simulink model "SpeedgoatCANOpen2Buses1ms"  (R2018b)
settings: Solver=ode8  StartTime=0.0  StopTime=inf  FixedStep=0.001  RelTol=1e-3  EnableMultiTasking=on
undefined symbols (not defined in the file or in its folder): DiscIntNeverNeededParam
libraries: slrtlib x6, speedgoatlib_IO691 x5, dspstat3 x5, simulink x5
(part 2 of 3)

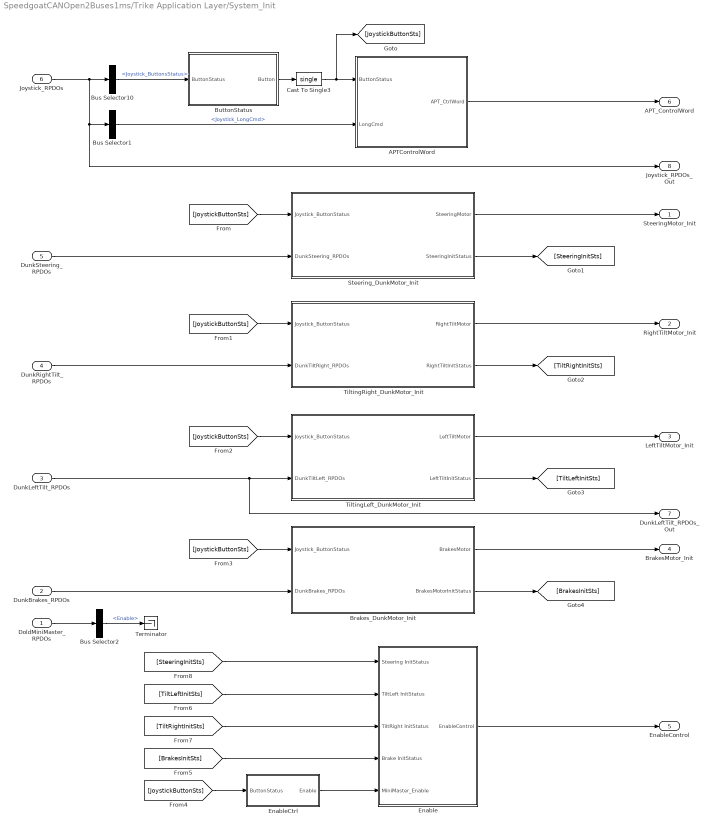
== system SpeedgoatCANOpen2Buses1ms/Trike Application Layer/System_Init ==
  DoldMiniMaster_RPDOs : Inport  OutDataTypeStr=Bus: Dold_RPDOs
  DunkBrakes_RPDOs : Inport  Port=2  OutDataTypeStr=Bus: Dunk_RPDOs
  DunkLeftTilt_RPDOs : Inport  Port=3  OutDataTypeStr=Bus: Dunk_RPDOs
  DunkRightTilt_RPDOs : Inport  Port=4  OutDataTypeStr=Bus: Dunk_RPDOs
  DunkSteering_RPDOs : Inport  Port=5  OutDataTypeStr=Bus: Dunk_RPDOs
  Joystick_RPDOs : Inport  Port=6  OutDataTypeStr=Bus: Joystick_RPDOs
  APTControlWord : MATLAB Function  TreatAsAtomicUnit=on
  Brakes_DunkMotor_Init : Subsystem
  Bus Selector1 : BusSelector  OutputSignals=Joystick_LongCmd
  Bus Selector10 : BusSelector  OutputSignals=Joystick_ButtonsStatus
  Bus Selector2 : BusSelector  OutputSignals=Enable
  ButtonStatus : MATLAB Function  TreatAsAtomicUnit=on
  Cast To Single3 : DataTypeConversion  OutDataTypeStr=single
  Enable : Subsystem
  EnableCtrl : Stateflow chart  TreatAsAtomicUnit=on
  Steering_DunkMotor_Init : Subsystem
  Terminator : Terminator
  TiltingLeft_DunkMotor_Init : Subsystem
  TiltingRight_DunkMotor_Init : Subsystem
  SteeringMotor_Init : Outport  OutDataTypeStr=Bus: Dunk_Init_TPDOs
  RightTiltMotor_Init : Outport  Port=2  OutDataTypeStr=Bus: Dunk_Init_TPDOs
  LeftTiltMotor_Init : Outport  Port=3  OutDataTypeStr=Bus: Dunk_Init_TPDOs
  BrakesMotor_Init : Outport  Port=4  OutDataTypeStr=Bus: DunkBrakes_Init_TPDOs
  EnableControl : Outport  Port=5
  APT_ControlWord : Outport  Port=6
  DunkLeftTilt_RPDOs_Out : Outport  Port=7  OutDataTypeStr=Bus: Dunk_RPDOs
  Joystick_RPDOs_Out : Outport  Port=8  OutDataTypeStr=Bus: Joystick_RPDOs
  wires:
  Bus Selector10/1 -> ButtonStatus/1(ButtonStatus)  "<Joystick_ButtonsStatus>"
  Joystick_RPDOs/1 -> Bus Selector10/1, Joystick_RPDOs_Out/1, Bus Selector1/1
  DunkBrakes_RPDOs/1 -> Brakes_DunkMotor_Init/2(DunkBrakes_RPDOs)
  DunkLeftTilt_RPDOs/1 -> TiltingLeft_DunkMotor_Init/2(DunkTiltLeft_RPDOs), DunkLeftTilt_RPDOs_Out/1
  DunkRightTilt_RPDOs/1 -> TiltingRight_DunkMotor_Init/2(DunkTiltRight_RPDOs)
  DunkSteering_RPDOs/1 -> Steering_DunkMotor_Init/2(DunkSteering_RPDOs)
  Steering_DunkMotor_Init/1(SteeringMotor) -> SteeringMotor_Init/1
  TiltingRight_DunkMotor_Init/1(RightTiltMotor) -> RightTiltMotor_Init/1
  TiltingLeft_DunkMotor_Init/1(LeftTiltMotor) -> LeftTiltMotor_Init/1
  Brakes_DunkMotor_Init/1(BrakesMotor) -> BrakesMotor_Init/1
  APTControlWord/1(APT_CtrlWord) -> APT_ControlWord/1
  Bus Selector1/1 -> APTControlWord/2(LongCmd)  "<Joystick_LongCmd>"
  ButtonStatus/1(Button) -> Cast To Single3/1
  Enable/1(EnableControl) -> EnableControl/1
  DoldMiniMaster_RPDOs/1 -> Bus Selector2/1
  EnableCtrl/1(Enable) -> Enable/5(MiniMaster_Enable)
  Bus Selector2/1 -> Terminator/1  "<Enable>"
  Cast To Single3/1 -> APTControlWord/1(ButtonStatus), [JoystickButtonSts]
  [JoystickButtonSts] -> Steering_DunkMotor_Init/1(Joystick_ButtonStatus)
  [JoystickButtonSts] -> TiltingRight_DunkMotor_Init/1(Joystick_ButtonStatus)
  [JoystickButtonSts] -> Brakes_DunkMotor_Init/1(Joystick_ButtonStatus)
  [JoystickButtonSts] -> TiltingLeft_DunkMotor_Init/1(Joystick_ButtonStatus)
  [JoystickButtonSts] -> EnableCtrl/1(ButtonStatus)
  [BrakesInitSts] -> Enable/4(Brake InitStatus)
  Brakes_DunkMotor_Init/2(BrakesMotorInitStatus) -> [BrakesInitSts]
  TiltingLeft_DunkMotor_Init/2(LeftTiltInitStatus) -> [TiltLeftInitSts]
  TiltingRight_DunkMotor_Init/2(RightTiltInitStatus) -> [TiltRightInitSts]
  Steering_DunkMotor_Init/2(SteeringInitStatus) -> [SteeringInitSts]
  [SteeringInitSts] -> Enable/1(Steering InitStatus)
  [TiltLeftInitSts] -> Enable/2(TiltLeft InitStatus)
  [TiltRightInitSts] -> Enable/3(TiltRight InitStatus)

== system SpeedgoatCANOpen2Buses1ms/Speedgoat_TPDOs/CAN Bus Communication/CANOpen Slave Protocol Stack - CAN Bus #1 (A) ==
  C Caller : CCaller  FunctionName=CANOpenSlave_ProcessStack  PortSpecificationStruct="%)30     .    ( D   8    (     @         %    \"     8    !     0         %  0 \"0    $    V    07)G3F%M90  4&]R=$YA;64 4V-O<&4     26YD97@     5'EP90      4VEZ90         .    ,     8    (    !          %    \"     $    $     0         0  0 <GA)1 X    P    !@    @    $          4    (     0    0    !         !  ! !R>$E$#@   #@    &    \"     0         !0    @    !    !0    $         $     4   !);G ...(+2763 chars)"
  CAN RX Wrapper : Subsystem
  CAN TX Wrapper : Subsystem
  wires:
  C Caller/2 -> CAN TX Wrapper/Enable, CAN TX Wrapper/2(DLC)
  CAN RX Wrapper/1(ID) -> C Caller/1
  C Caller/1 -> CAN TX Wrapper/1(ID)
  CAN RX Wrapper/2(DLC) -> C Caller/2
  C Caller/3 -> CAN TX Wrapper/3(DATA)
  CAN RX Wrapper/3(DATA) -> C Caller/3

== system SpeedgoatCANOpen2Buses1ms/Speedgoat_TPDOs/CAN Bus Communication/CANOpen Slave Protocol Stack - CAN Bus #2 (B) ==
  C Caller : CCaller  FunctionName=CANOpenSlave_ProcessStack_APT  PortSpecificationStruct="%)30     .    ( D   8    (     @         %    \"     8    !     0         %  0 \"0    $    V    07)G3F%M90  4&]R=$YA;64 4V-O<&4     26YD97@     5'EP90      4VEZ90         .    ,     8    (    !          %    \"     $    $     0         0  0 <GA)1 X    P    !@    @    $          4    (     0    0    !         !  ! !R>$E$#@   #@    &    \"     0         !0    @    !    !0    $         $     4   !);G ...(+2763 chars)"
  CAN RX Wrapper : Subsystem
  CAN TX Wrapper : Subsystem
  wires:
  CAN RX Wrapper/3(DATA) -> C Caller/3
  C Caller/3 -> CAN TX Wrapper/3(DATA)
  CAN RX Wrapper/2(DLC) -> C Caller/2
  C Caller/1 -> CAN TX Wrapper/1(ID)
  CAN RX Wrapper/1(ID) -> C Caller/1
  C Caller/2 -> CAN TX Wrapper/2(DLC), CAN TX Wrapper/Enable

== system SpeedgoatCANOpen2Buses1ms/Trike Application Layer/System_Control/BrakeControl ==
  VehSpeed_SI [m/s] : Inport
  DriverBrakingRequest : Inport  Port=2
  Joystick_LongCmd : Inport  Port=3
  Joystick_ButtonStatus : Inport  Port=4
  BrakesMotor_CurrentInit : Inport  Port=5
  BrakeCtrlIn : Inport  Port=6
  Cast To Single3 : DataTypeConversion  Commented=on  OutDataTypeStr=single
  DecisionBrakeCtrl : Stateflow chart  TreatAsAtomicUnit=on
  Gain4 : Gain  Commented=on  Gain=0.001
  Gain5 : Gain  Gain=-1
  MATLAB Function : MATLAB Function  Commented=on  TreatAsAtomicUnit=on
  Subsystem : Subsystem
  Sum4 : Sum  Inputs=|++
  BrakesMotor_CurrentReq [mA] : Outport
  BrakesMotor_BrakeCtrl : Outport  Port=2
  wires:
  Joystick_LongCmd/1 -> DecisionBrakeCtrl/5(JsLongCmd)
  MATLAB Function/1(button) -> Cast To Single3/1
  Joystick_ButtonStatus/1 -> DecisionBrakeCtrl/4(JsButton)
  Cast To Single3/1 -> Gain4/1
  BrakesMotor_CurrentInit/1 -> Gain5/1
  Gain5/1 -> Sum4/1  "BrakesMotor_CurrentInit [mA]"
  Sum4/1 -> BrakesMotor_CurrentReq [mA]/1
  BrakeCtrlIn/1 -> DecisionBrakeCtrl/3(BrakeCtrlIn)
  DecisionBrakeCtrl/2(BrakeCtrl) -> BrakesMotor_BrakeCtrl/1
  DriverBrakingRequest/1 -> Subsystem/1(BrakingRequest)  "BrakingRequest [LSB]"
  Subsystem/1(BrakesMotor_CurrentReq) -> DecisionBrakeCtrl/1(BrakesMotor_CurrentReqIn)
  VehSpeed_SI [m/s]/1 -> DecisionBrakeCtrl/2(VehSpeed)
  DecisionBrakeCtrl/1(BrakesMotor_CurrentReq) -> Sum4/2  "Retract_current"

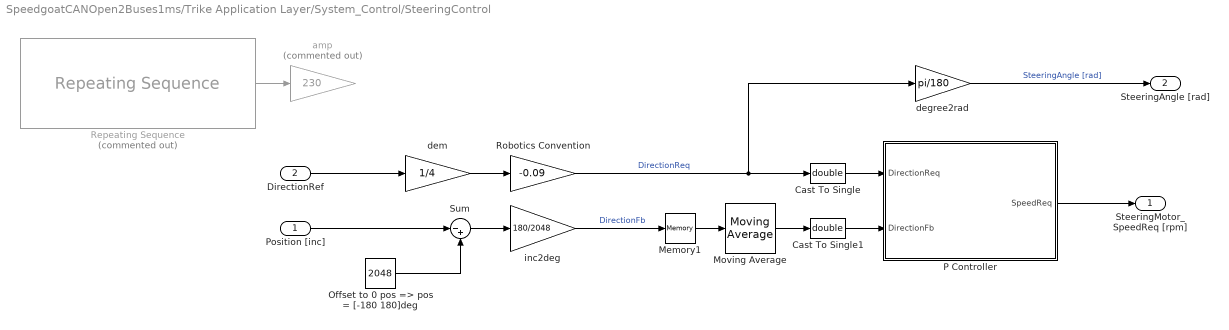
== system SpeedgoatCANOpen2Buses1ms/Trike Application Layer/System_Control/SteeringControl ==
  Position [inc] : Inport
  DirectionRef : Inport  Port=2
  Cast To Single : DataTypeConversion  OutDataTypeStr=double
  Cast To Single1 : DataTypeConversion  OutDataTypeStr=double
  Memory1 : Memory  InheritSampleTime=on
  Moving Average : dspstat3/Moving Average  Method=Sliding window  ForgettingFactorPort=off  SpecifyWindowLength=on  WindowLength=1  ForgettingFactor=0.9  SimulateUsing=Code generation
  Offset to 0 pos => pos = [-180 180]deg : Constant  Value=2048
  P Controller : MATLAB Function  TreatAsAtomicUnit=on  SystemSampleTime=5e-3
  Repeating Sequence : simulink/Sources/Repeating Sequence  Commented=on  rep_seq_t=[0 3 3.01 6 6.01 9 9.01 12]*5  rep_seq_y=[1 1 0 0 -1 -1 0 0]
  Robotics Convention : Gain  Gain=-0.09
  Sum : Sum  Inputs=|-+
  amp : Gain  Commented=on  Gain=230
  degree2rad : Gain  Gain=pi/180
  dem : Gain  Gain=1/4
  inc2deg : Gain  Gain=180/2048
  SteeringMotor_SpeedReq [rpm] : Outport
  SteeringAngle [rad] : Outport  Port=2
  wires:
  Memory1/1 -> Moving Average/1
  degree2rad/1 -> SteeringAngle [rad]/1  "SteeringAngle [rad]"
  inc2deg/1 -> Memory1/1  "DirectionFb"
  DirectionRef/1 -> dem/1
  P Controller/1(SpeedReq) -> SteeringMotor_SpeedReq [rpm]/1
  Robotics Convention/1 -> Cast To Single/1, degree2rad/1  "DirectionReq"
  Cast To Single/1 -> P Controller/1(DirectionReq)
  Cast To Single1/1 -> P Controller/2(DirectionFb)
  Position [inc]/1 -> Sum/1
  Sum/1 -> inc2deg/1
  Offset to 0 pos => pos = [-180 180]deg/1 -> Sum/2
  Moving Average/1 -> Cast To Single1/1
  Repeating Sequence/1 -> amp/1
  dem/1 -> Robotics Convention/1

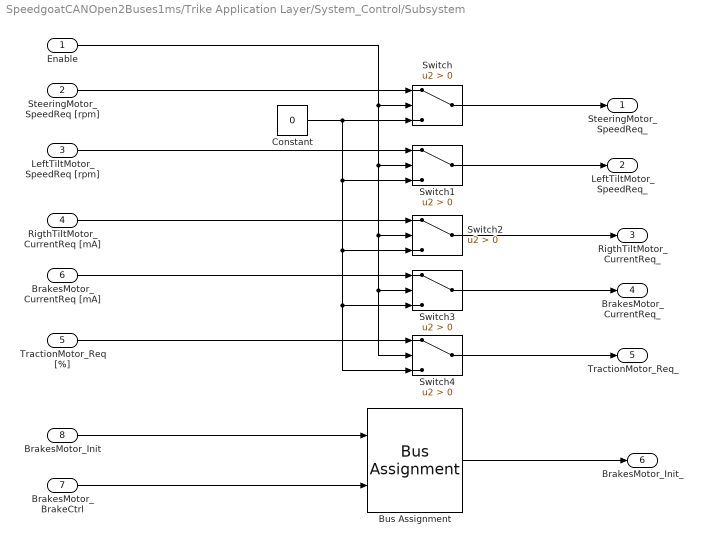
== system SpeedgoatCANOpen2Buses1ms/Trike Application Layer/System_Control/Subsystem ==
  Enable : Inport
  SteeringMotor_SpeedReq [rpm] : Inport  Port=2
  LeftTiltMotor_SpeedReq [rpm] : Inport  Port=3
  RigthTiltMotor_CurrentReq [mA] : Inport  Port=4
  TractionMotor_Req [%] : Inport  Port=5
  BrakesMotor_CurrentReq [mA] : Inport  Port=6
  BrakesMotor_BrakeCtrl : Inport  Port=7
  BrakesMotor_Init : Inport  Port=8  OutDataTypeStr=Bus: DunkBrakes_Init_TPDOs
  Bus Assignment : BusAssignment  AssignedSignals=BrakeCtrl
  Constant : Constant  Value=0
  Switch{,1..4} (5 alike) : Switch  Criteria=u2 > Threshold
  SteeringMotor_SpeedReq_ : Outport
  LeftTiltMotor_SpeedReq_ : Outport  Port=2
  RigthTiltMotor_CurrentReq_ : Outport  Port=3
  BrakesMotor_CurrentReq_ : Outport  Port=4
  TractionMotor_Req_ : Outport  Port=5
  BrakesMotor_Init_ : Outport  Port=6  OutDataTypeStr=Bus: DunkBrakes_Init_TPDOs
  wires:
  TractionMotor_Req [%]/1 -> Switch4/1
  Switch1/1 -> LeftTiltMotor_SpeedReq_/1
  Switch2/1 -> RigthTiltMotor_CurrentReq_/1
  Enable/1 -> Switch1/2, Switch2/2, Switch3/2, Switch4/2, Switch/2
  SteeringMotor_SpeedReq [rpm]/1 -> Switch/1
  LeftTiltMotor_SpeedReq [rpm]/1 -> Switch1/1
  Constant/1 -> Switch3/3, Switch4/3, Switch2/3, Switch1/3, Switch/3
  Switch/1 -> SteeringMotor_SpeedReq_/1
  BrakesMotor_CurrentReq [mA]/1 -> Switch3/1
  Switch3/1 -> BrakesMotor_CurrentReq_/1
  Switch4/1 -> TractionMotor_Req_/1
  RigthTiltMotor_CurrentReq [mA]/1 -> Switch2/1
  Bus Assignment/1 -> BrakesMotor_Init_/1
  BrakesMotor_Init/1 -> Bus Assignment/1
  BrakesMotor_BrakeCtrl/1 -> Bus Assignment/2

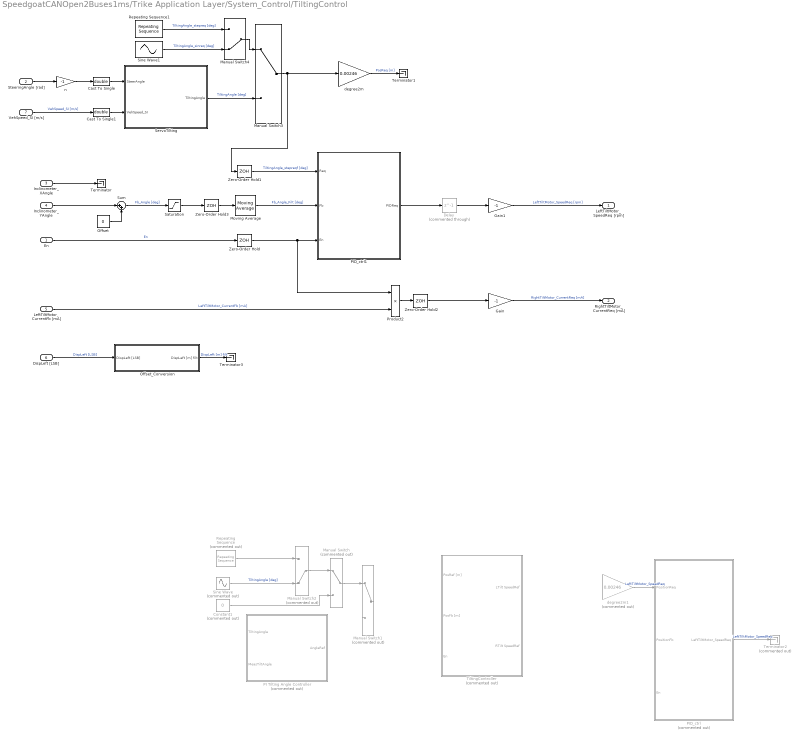
== system SpeedgoatCANOpen2Buses1ms/Trike Application Layer/System_Control/TiltingControl ==
  En : Inport
  SteeringAngle [rad] : Inport  Port=2
  Inclinometer_XAngle : Inport  Port=3
  Inclinometer_YAngle : Inport  Port=4
  LeftTiltMotor_CurrentFb [mA] : Inport  Port=5
  DispLeft [LSB] : Inport  Port=6
  VehSpeed_SI [m/s] : Inport  Port=7
  Cast To Single : DataTypeConversion  OutDataTypeStr=double
  Cast To Single1 : DataTypeConversion  OutDataTypeStr=double
  Constant1 : Constant  Commented=on  Value=0
  Delay : Delay  Commented=through  DelayLength=1  SampleTime=0.005
  Gain : Gain  Gain=-1
  Gain1 : Gain  Gain=-1
  Manual Switch : ManualSwitch  Commented=on
  Manual Switch1 : ManualSwitch  Commented=on
  Manual Switch2 : ManualSwitch  Commented=on  CurrentSetting=0
  Manual Switch3 : ManualSwitch
  Manual Switch4 : ManualSwitch  CurrentSetting=0
  Moving Average : dspstat3/Moving Average  Method=Sliding window  ForgettingFactorPort=off  SpecifyWindowLength=on  WindowLength=10  ForgettingFactor=0.9  SimulateUsing=Code generation
  Offset : Constant  Value=0
  Offset_Conversion : Subsystem
  PI Tilting Angle Controller : Subsystem  Commented=on  TreatAsAtomicUnit=on  SystemSampleTime=10e-3
  PID_ctrl : Subsystem  Commented=on  mask{Kp=80000, Ki=200, Kd=0, Ts=0.005, N=1, FF_En=0, Req_lim=2000}
      mask prompts: N "FilterOrder"; FF_En "FeedForward En"; Req_lim "Req_sat"
  PID_ctrl1 : Subsystem  mask{Kp=90, Ki=0, Kd=2, Ts=0.015, N=4, FF_En=0, Req_lim=1000}
      mask prompts: N "FilterOrder"; FF_En "FeedForward En"; Req_lim "Req_sat"
  Product2 : Product
  Repeating Sequence : simulink/Sources/Repeating Sequence  Commented=on  rep_seq_t=[0 3 3.01 6 6.01 9 9.01 12]*5  rep_seq_y=[ 0 0 1 1 0 0 1 1]*3
  Repeating Sequence1 : simulink/Sources/Repeating Sequence  rep_seq_t=[0 3 3.001 6 6.001 9 9.001 12] * 4 + 50  rep_seq_y=[ 0 0 1 1 0 0 -1 -1]*2
  Saturation : Saturate  UpperLimit=30  LowerLimit=-30
  ServoTilting : MATLAB Function  TreatAsAtomicUnit=on
      settings: MinAlgLoopOccurrences=on
  Sine Wave : Sin  Commented=on  Amplitude=2  Frequency=0.5  SampleTime=0
  Sine Wave1 : Sin  Amplitude=2  Frequency=0.5  SampleTime=0
  Sum : Sum  Inputs=|++
  Terminator : Terminator
  Terminator1 : Terminator
  Terminator2 : Terminator  Commented=on
  Terminator3 : Terminator
  TiltingController : Subsystem  Commented=on  VariantControlMode=Label  Variant=on  VariantControl=Variant1  LabelModeActiveChoice=V1  PropagateVariantConditions=on
  Zero-Order Hold{,1..3} (4 alike) : ZeroOrderHold  SampleTime=0.005
  degree2m : Gain  Gain=0.00246
  degree2m1 : Gain  Commented=on  Gain=0.00246
  n : Gain  Gain=-1
  LeftTiltMotor_SpeedReq [rpm] : Outport
  RightTiltMotor_CurrentReq [mA] : Outport  Port=2
  wires:
  SteeringAngle [rad]/1 -> n/1
  Cast To Single/1 -> ServoTilting/1(SteerAngle)
  Cast To Single1/1 -> ServoTilting/2(VehSpeed_SI)
  VehSpeed_SI [m/s]/1 -> Cast To Single1/1  "VehSpeed_SI [m/s]"
  Constant1/1 -> Manual Switch/2
  ServoTilting/1(TiltingAngle) -> Manual Switch3/2  "TiltingAngle [deg]"
  Manual Switch/1 -> Manual Switch1/1
  n/1 -> Cast To Single/1
  Sine Wave/1 -> Manual Switch2/2  "TiltingAngle [deg]"
  En/1 -> Zero-Order Hold/1  "En"
  Offset_Conversion/1(DispLeft [m] filt) -> Terminator3/1  "DispLeft [m] filt"
  DispLeft [LSB]/1 -> Offset_Conversion/1(DispLeft [LSB])  "DispLeft [LSB]"
  Repeating Sequence/1 -> Manual Switch2/1
  Manual Switch2/1 -> Manual Switch/1
  degree2m/1 -> Terminator1/1  "PosReq [m]"
  degree2m1/1 -> PID_ctrl/1(PositionReq)  "LeftTiltMotor_SpeedReq"
  LeftTiltMotor_CurrentFb [mA]/1 -> Product2/2  "LeftTiltMotor_CurrentFb [mA]"
  Gain/1 -> RightTiltMotor_CurrentReq [mA]/1  "RightTiltMotor_CurrentReq [mA]"
  Product2/1 -> Zero-Order Hold2/1
  Inclinometer_XAngle/1 -> Terminator/1
  Sine Wave1/1 -> Manual Switch4/2  "TiltingAngle_sinreq [deg]"
  Moving Average/1 -> PID_ctrl1/2(Fb)  "Fb_Angle_Filt [deg]"
  Offset/1 -> Sum/2
  Saturation/1 -> Zero-Order Hold3/1
  Sum/1 -> Saturation/1  "Fb_Angle [deg]"
  Manual Switch3/1 -> Zero-Order Hold1/1, degree2m/1
  PID_ctrl/1(LeftTiltMotor_SpeedReq) -> Terminator2/1  "LeftTiltMotor_SpeedReq"
  Gain1/1 -> LeftTiltMotor_SpeedReq [rpm]/1  "LeftTiltMotor_SpeedReq [rpm]"
  Repeating Sequence1/1 -> Manual Switch4/1  "TiltingAngle_stepreq [deg]"
  Manual Switch4/1 -> Manual Switch3/1
  Zero-Order Hold1/1 -> PID_ctrl1/1(Req)  "TiltingAngle_stepreqf [deg]"
  Inclinometer_YAngle/1 -> Sum/1
  Zero-Order Hold/1 -> Product2/1, PID_ctrl1/3(En)
  PID_ctrl1/1(PIDReq) -> Delay/1
  Zero-Order Hold2/1 -> Gain/1
  Delay/1 -> Gain1/1
  Zero-Order Hold3/1 -> Moving Average/1

== system SpeedgoatCANOpen2Buses1ms/Trike Application Layer/System_Control/TractionControl ==
  Driver_TorqueReq [%] : Inport
  VehSpeed_Fb : Inport  Port=2
  Abs : Abs
  Cast To Single1 : DataTypeConversion
  Cast To Single2 : DataTypeConversion
  Cast To Single3 : DataTypeConversion
  Gain1 : Gain  Gain=1/10
  Gain2 : Gain  Gain=pi/30
  Terminator1 : Terminator
  WheelRadius : Gain  Gain=0.25
  m/s2Km/h : Gain  Gain=3.6
  VehSpeed_SI [m/s] : Outport
  TractionReq [%] : Outport  Port=2
  wires:
  Driver_TorqueReq [%]/1 -> Cast To Single1/1
  Abs/1 -> TractionReq [%]/1  "TractionReq"
  WheelRadius/1 -> m/s2Km/h/1, Cast To Single2/1  "VehSpeed_SI"
  VehSpeed_Fb/1 -> Cast To Single3/1
  Gain2/1 -> WheelRadius/1  "Speed_SI"
  m/s2Km/h/1 -> Terminator1/1  "VehSpeed_Km/h"
  Gain1/1 -> Abs/1
  Cast To Single3/1 -> Gain2/1
  Cast To Single1/1 -> Gain1/1
  Cast To Single2/1 -> VehSpeed_SI [m/s]/1

== system SpeedgoatCANOpen2Buses1ms/Trike Application Layer/System_Init/Brakes_DunkMotor_Init ==
  Joystick_ButtonStatus : Inport
  DunkBrakes_RPDOs : Inport  Port=2  OutDataTypeStr=Bus: Dunk_RPDOs
  Bus Creator : BusCreator  Inputs=5  OutDataTypeStr=Bus: DunkBrakes_Init_TPDOs
  Bus Selector1 : BusSelector  OutputSignals=DunkD_ActualVelocity
  Cast To Single{,1..3} (4 alike) : DataTypeConversion  OutDataTypeStr=uint8
  Cast To Single4 : DataTypeConversion  OutDataTypeStr=int16
  Constant : Constant  OutDataTypeStr=single
  DunkD_Brake_Init_CurrentMode : Stateflow chart  TreatAsAtomicUnit=on
  Terminator : Terminator
  BrakesMotor : Outport  OutDataTypeStr=Bus: DunkBrakes_Init_TPDOs
  BrakesMotorInitStatus : Outport  Port=2
  wires:
  DunkBrakes_RPDOs/1 -> Bus Selector1/1
  Bus Creator/1 -> BrakesMotor/1
  Cast To Single1/1 -> Bus Creator/1  "ClearError"
  Cast To Single/1 -> Bus Creator/2  "DeviceMode"
  Cast To Single2/1 -> Bus Creator/3  "BrakeCtrl"
  Cast To Single3/1 -> Bus Creator/4  "PowerEnable"
  DunkD_Brake_Init_CurrentMode/6(InitStatus) -> BrakesMotorInitStatus/1
  DunkD_Brake_Init_CurrentMode/1(ClearError) -> Cast To Single1/1
  Joystick_ButtonStatus/1 -> DunkD_Brake_Init_CurrentMode/1(ButtonStatus)
  DunkD_Brake_Init_CurrentMode/2(DeviceMode) -> Cast To Single/1
  DunkD_Brake_Init_CurrentMode/3(BrakeCtrl) -> Cast To Single2/1
  DunkD_Brake_Init_CurrentMode/4(PowerEnable) -> Cast To Single3/1
  Constant/1 -> DunkD_Brake_Init_CurrentMode/2(ReadError)
  Bus Selector1/1 -> Terminator/1  "<DunkD_ActualVelocity>"
  DunkD_Brake_Init_CurrentMode/5(BrakesMotor_CurrentInit) -> Cast To Single4/1
  Cast To Single4/1 -> Bus Creator/5  "CurrentInit"

== system SpeedgoatCANOpen2Buses1ms/Trike Application Layer/System_Init/Enable ==
  Steering InitStatus : Inport
  TiltLeft InitStatus : Inport  Port=2
  TiltRight InitStatus : Inport  Port=3
  Brake InitStatus : Inport  Port=4
  MiniMaster_Enable : Inport  Port=5
  Compare To Constant : simulink/Logic and Bit Operations/Compare To Constant  relop===  const=5  OutDataTypeStr=boolean
  Sum : Sum  Inputs=+++++
  EnableControl : Outport
  wires:
  Sum/1 -> Compare To Constant/1
  Brake InitStatus/1 -> Sum/4  "Brake_InitStatus"
  Steering InitStatus/1 -> Sum/1  "Steering_InitStatus"
  TiltRight InitStatus/1 -> Sum/3  "TiltRight_InitStatus"
  TiltLeft InitStatus/1 -> Sum/2  "TiltLeft_InitStatus"
  MiniMaster_Enable/1 -> Sum/5  "MiniMaster_Enable"
  Compare To Constant/1 -> EnableControl/1  "EnableControl"

== system SpeedgoatCANOpen2Buses1ms/Trike Application Layer/System_Init/Steering_DunkMotor_Init ==
  Joystick_ButtonStatus : Inport
  DunkSteering_RPDOs : Inport  Port=2  OutDataTypeStr=Bus: Dunk_RPDOs
  Bus Creator : BusCreator  Inputs=4  OutDataTypeStr=Bus: Dunk_Init_TPDOs
  Bus Selector1 : BusSelector  OutputSignals=DunkA_ActualVelocity
  Cast To Single{,1..3} (4 alike) : DataTypeConversion  OutDataTypeStr=uint8
  Constant : Constant  OutDataTypeStr=single
  DunkA_Steering_Init_SpeedMode : Stateflow chart  TreatAsAtomicUnit=on
  Terminator : Terminator
  SteeringMotor : Outport  OutDataTypeStr=Bus: Dunk_Init_TPDOs
  SteeringInitStatus : Outport  Port=2
  wires:
  Bus Creator/1 -> SteeringMotor/1
  DunkSteering_RPDOs/1 -> Bus Selector1/1
  DunkA_Steering_Init_SpeedMode/1(ClearError) -> Cast To Single1/1
  DunkA_Steering_Init_SpeedMode/2(DeviceMode) -> Cast To Single/1
  DunkA_Steering_Init_SpeedMode/3(BrakeCtrl) -> Cast To Single2/1
  DunkA_Steering_Init_SpeedMode/4(PowerEnable) -> Cast To Single3/1
  Joystick_ButtonStatus/1 -> DunkA_Steering_Init_SpeedMode/1(ButtonStatus)
  Constant/1 -> DunkA_Steering_Init_SpeedMode/2(ReadError)
  Cast To Single1/1 -> Bus Creator/1  "ClearError"
  Cast To Single/1 -> Bus Creator/2  "DeviceMode"
  Cast To Single2/1 -> Bus Creator/3  "BrakeCtrl"
  Cast To Single3/1 -> Bus Creator/4  "PowerEnable"
  DunkA_Steering_Init_SpeedMode/5(InitStatus) -> SteeringInitStatus/1
  Bus Selector1/1 -> Terminator/1  "<DunkA_ActualVelocity>"

== system SpeedgoatCANOpen2Buses1ms/Trike Application Layer/System_Init/TiltingLeft_DunkMotor_Init ==
  Joystick_ButtonStatus : Inport
  DunkTiltLeft_RPDOs : Inport  Port=2  OutDataTypeStr=Bus: Dunk_RPDOs
  Bus Creator : BusCreator  Inputs=4  OutDataTypeStr=Bus: Dunk_Init_TPDOs
  Bus Selector1 : BusSelector  OutputSignals=DunkC_ActualCurrent
  Cast To Single{,1..3} (4 alike) : DataTypeConversion  OutDataTypeStr=uint8
  Constant : Constant  OutDataTypeStr=single
  DunkC_TiltLeft_Init_CurrentMode : Stateflow chart  TreatAsAtomicUnit=on
  Terminator : Terminator
  LeftTiltMotor : Outport  OutDataTypeStr=Bus: Dunk_Init_TPDOs
  LeftTiltInitStatus : Outport  Port=2
  wires:
  Bus Creator/1 -> LeftTiltMotor/1
  DunkTiltLeft_RPDOs/1 -> Bus Selector1/1
  Cast To Single1/1 -> Bus Creator/1  "ClearError"
  Cast To Single/1 -> Bus Creator/2  "DeviceMode"
  Cast To Single2/1 -> Bus Creator/3  "BrakeCtrl"
  Cast To Single3/1 -> Bus Creator/4  "PowerEnable"
  DunkC_TiltLeft_Init_CurrentMode/5(InitStatus) -> LeftTiltInitStatus/1
  DunkC_TiltLeft_Init_CurrentMode/1(ClearError) -> Cast To Single1/1
  Joystick_ButtonStatus/1 -> DunkC_TiltLeft_Init_CurrentMode/1(ButtonStatus)
  DunkC_TiltLeft_Init_CurrentMode/2(DeviceMode) -> Cast To Single/1
  DunkC_TiltLeft_Init_CurrentMode/3(BrakeCtrl) -> Cast To Single2/1
  DunkC_TiltLeft_Init_CurrentMode/4(PowerEnable) -> Cast To Single3/1
  Constant/1 -> DunkC_TiltLeft_Init_CurrentMode/2(ReadError)
  Bus Selector1/1 -> Terminator/1  "<DunkC_ActualCurrent>"

== system SpeedgoatCANOpen2Buses1ms/Trike Application Layer/System_Init/TiltingRight_DunkMotor_Init ==
  Joystick_ButtonStatus : Inport
  DunkTiltRight_RPDOs : Inport  Port=2  OutDataTypeStr=Bus: Dunk_RPDOs
  Bus Creator : BusCreator  Inputs=4  OutDataTypeStr=Bus: Dunk_Init_TPDOs
  Bus Selector1 : BusSelector  OutputSignals=DunkB_ActualCurrent
  Cast To Single{,1..3} (4 alike) : DataTypeConversion  OutDataTypeStr=uint8
  Constant : Constant  OutDataTypeStr=single
  DunkB_TiltRight_Init_CurrentMode : Stateflow chart  TreatAsAtomicUnit=on
  Terminator : Terminator
  RightTiltMotor : Outport  OutDataTypeStr=Bus: Dunk_Init_TPDOs
  RightTiltInitStatus : Outport  Port=2
  wires:
  DunkTiltRight_RPDOs/1 -> Bus Selector1/1
  Bus Creator/1 -> RightTiltMotor/1
  DunkB_TiltRight_Init_CurrentMode/5(InitStatus) -> RightTiltInitStatus/1
  Cast To Single/1 -> Bus Creator/2  "DeviceMode"
  Constant/1 -> DunkB_TiltRight_Init_CurrentMode/2(ReadError)
  Cast To Single2/1 -> Bus Creator/3  "BrakeCtrl"
  DunkB_TiltRight_Init_CurrentMode/4(PowerEnable) -> Cast To Single3/1
  DunkB_TiltRight_Init_CurrentMode/3(BrakeCtrl) -> Cast To Single2/1
  Cast To Single3/1 -> Bus Creator/4  "PowerEnable"
  DunkB_TiltRight_Init_CurrentMode/2(DeviceMode) -> Cast To Single/1
  Cast To Single1/1 -> Bus Creator/1  "ClearError"
  DunkB_TiltRight_Init_CurrentMode/1(ClearError) -> Cast To Single1/1
  Joystick_ButtonStatus/1 -> DunkB_TiltRight_Init_CurrentMode/1(ButtonStatus)
  Bus Selector1/1 -> Terminator/1  "<DunkB_ActualCurrent>"

== system SpeedgoatCANOpen2Buses1ms/Speedgoat_TPDOs/CAN Bus Communication/CANOpen Slave Protocol Stack - CAN Bus #1 (A)/CAN RX Wrapper ==
  CAN Read : speedgoatlib_IO691/CAN Read  id=1  ts=Ts  channel=1  messageType=RAW  canType=CAN (HS)  initValues=[691 1 0.0001 0 2 1]
      settings: SourceProductName=Simulink Real-Time: Speedgoat Library
  Constant : Constant  Commented=on  Value=0  OutDataTypeStr=Inherit: Inherit via back propagation
  Switch : Switch  Criteria=u2 > Threshold
  Terminator : Terminator
  Terminator1 : Terminator
  ID : Outport
  DLC : Outport  Port=2
  DATA : Outport  Port=3
  wires:
  CAN Read/4 -> Switch/3
  CAN Read/5 -> Terminator1/1
  Switch/1 -> DLC/1
  CAN Read/2 -> ID/1
  CAN Read/3 -> Switch/2
  CAN Read/6 -> DATA/1
  Constant/1 -> Switch/1
  CAN Read/1 -> Terminator/1

== system SpeedgoatCANOpen2Buses1ms/Speedgoat_TPDOs/CAN Bus Communication/CANOpen Slave Protocol Stack - CAN Bus #1 (A)/CAN TX Wrapper ==
  ID : Inport
  DLC : Inport  Port=2
  DATA : Inport  Port=3
  Enable : EnablePort
  CAN Write : speedgoatlib_IO691/CAN Write  id=1  ts=Ts  channel=1  messageType=RAW  enableStatusPort=off  canType=CAN (HS)  initValues=[691 1 0.0001 0 2 1 0]
      settings: SourceProductName=Simulink Real-Time: Speedgoat Library
  Constant : Constant  Value=0  OutDataTypeStr=Inherit: Inherit via back propagation
  wires:
  ID/1 -> CAN Write/1
  DATA/1 -> CAN Write/4
  DLC/1 -> CAN Write/3
  Constant/1 -> CAN Write/2

== system SpeedgoatCANOpen2Buses1ms/Speedgoat_TPDOs/CAN Bus Communication/CANOpen Slave Protocol Stack - CAN Bus #2 (B)/CAN RX Wrapper ==
  CAN Read : speedgoatlib_IO691/CAN Read  id=1  ts=Ts  channel=2  messageType=RAW  canType=CAN (HS)  initValues=[691 1 0.0001 1 2 1]
      settings: SourceProductName=Simulink Real-Time: Speedgoat Library
  Constant : Constant  Commented=on  Value=0  OutDataTypeStr=Inherit: Inherit via back propagation
  Switch : Switch  Criteria=u2 > Threshold
  Terminator : Terminator
  Terminator1 : Terminator
  ID : Outport
  DLC : Outport  Port=2
  DATA : Outport  Port=3
  wires:
  CAN Read/1 -> Terminator/1
  Constant/1 -> Switch/1
  CAN Read/6 -> DATA/1
  CAN Read/3 -> Switch/2
  CAN Read/2 -> ID/1
  Switch/1 -> DLC/1
  CAN Read/5 -> Terminator1/1
  CAN Read/4 -> Switch/3

== system SpeedgoatCANOpen2Buses1ms/Speedgoat_TPDOs/CAN Bus Communication/CANOpen Slave Protocol Stack - CAN Bus #2 (B)/CAN TX Wrapper ==
  ID : Inport
  DLC : Inport  Port=2
  DATA : Inport  Port=3
  Enable : EnablePort
  CAN Write : speedgoatlib_IO691/CAN Write  id=1  ts=Ts  channel=2  messageType=RAW  enableStatusPort=off  canType=CAN (HS)  initValues=[691 1 0.0001 1 2 1 0]
      settings: SourceProductName=Simulink Real-Time: Speedgoat Library
  Constant : Constant  Value=0  OutDataTypeStr=Inherit: Inherit via back propagation
  wires:
  Constant/1 -> CAN Write/2
  DLC/1 -> CAN Write/3
  DATA/1 -> CAN Write/4
  ID/1 -> CAN Write/1

== system SpeedgoatCANOpen2Buses1ms/Trike Application Layer/System_Control/BrakeControl/Subsystem ==
  BrakingRequest : Inport
  Amp2mAmp : Gain  Gain=1000
  Data Type Conversion : DataTypeConversion  OutDataTypeStr=uint16
  Data Type Conversion1 : DataTypeConversion  OutDataTypeStr=single
  Delay : Delay
  Gain1 : Gain  Gain=12.7
  Gain2 : Gain  Gain=-1
  GetInPercent : Gain  Gain=0.00015625
  Retract : Stateflow chart  TreatAsAtomicUnit=on
  Saturation : Saturate  UpperLimit=0  LowerLimit=-1
  Saturation1 : Saturate  UpperLimit=10000  LowerLimit=3600
  Saturation2 : Saturate  UpperLimit=12  LowerLimit=-12
  Sum : Sum  Inputs=|+-
  Sum1 : Sum  Inputs=|+-
  Sum2 : Sum  Inputs=|++
  offset : Constant  Value=3600
  BrakesMotor_CurrentReq : Outport
  wires:
  Saturation1/1 -> Sum/1
  Gain1/1 -> Sum2/1
  Gain2/1 -> Saturation/1
  Sum1/1 -> Retract/1(PedalTravelGradient)
  GetInPercent/1 -> Gain2/1, Data Type Conversion1/1  "br_percent2"
  Data Type Conversion/1 -> Saturation1/1
  Retract/1(Br_CurrentReq) -> Sum2/2  "Retract_current"
  Saturation2/1 -> Amp2mAmp/1
  Data Type Conversion1/1 -> Delay/1, Sum1/2, Retract/2(PedalTravel)
  Sum2/1 -> Saturation2/1
  Sum/1 -> GetInPercent/1
  Delay/1 -> Sum1/1
  offset/1 -> Sum/2
  Saturation/1 -> Gain1/1
  BrakingRequest/1 -> Data Type Conversion/1
  Amp2mAmp/1 -> BrakesMotor_CurrentReq/1  "BrakesMotor_CurrentReq"

== system SpeedgoatCANOpen2Buses1ms/Trike Application Layer/System_Control/TiltingControl/Offset_Conversion ==
  DispLeft [LSB] : Inport
  Discrete Filter : DiscreteFilter  Numerator=[0.0201 0.0402 0.0201]  Denominator=[1 -1.561 0.6414]  SampleTime=0.005
  LSB2Volt : Gain  Gain=5/16380
  Memory1 : Memory  InheritSampleTime=on
  Offset for 0 deg : Constant  Value=3.34249
  Sum : Sum  Inputs=|+-
  Volt2meter : Gain  Gain=0.076/5
  DispLeft [m] filt : Outport
  wires:
  Volt2meter/1 -> Discrete Filter/1  "DispLeft [m]"
  Offset for 0 deg/1 -> Sum/2
  Sum/1 -> Volt2meter/1  "DispLeftOffset [Volt]"
  LSB2Volt/1 -> Sum/1  "DispLeft [Volt]"
  Discrete Filter/1 -> Memory1/1
  Memory1/1 -> DispLeft [m] filt/1
  DispLeft [LSB]/1 -> LSB2Volt/1

== system SpeedgoatCANOpen2Buses1ms/Trike Application Layer/System_Control/TiltingControl/PI Tilting Angle Controller ==
  TiltingAngle : Inport
  MeasTiltAngle : Inport  Port=2
  Discrete-Time Integrator : DiscreteIntegrator  IntegratorMethod=Integration: Trapezoidal  SampleTime=-1  ICPrevOutput=DiscIntNeverNeededParam  ICPrevScaledInput=DiscIntNeverNeededParam
  FeedbackP_tilt : Gain  Gain=0.1
  FeedbackP_tilt1 : Gain  Gain=100 * 10e-3
  Gain1 : Gain  Gain=-1
  Sum1 : Sum  Inputs=|+-
  Sum3 : Sum  Inputs=|++
  Zero-Order Hold : ZeroOrderHold  SampleTime=-1
  AngleRef : Outport
  wires:
  Zero-Order Hold/1 -> Discrete-Time Integrator/1
  Sum1/1 -> FeedbackP_tilt/1, FeedbackP_tilt1/1
  MeasTiltAngle/1 -> Sum1/2  "MeasTiltAngle"
  FeedbackP_tilt/1 -> Sum3/1
  FeedbackP_tilt1/1 -> Zero-Order Hold/1
  Discrete-Time Integrator/1 -> Sum3/2
  TiltingAngle/1 -> Sum1/1
  Sum3/1 -> Gain1/1
  Gain1/1 -> AngleRef/1

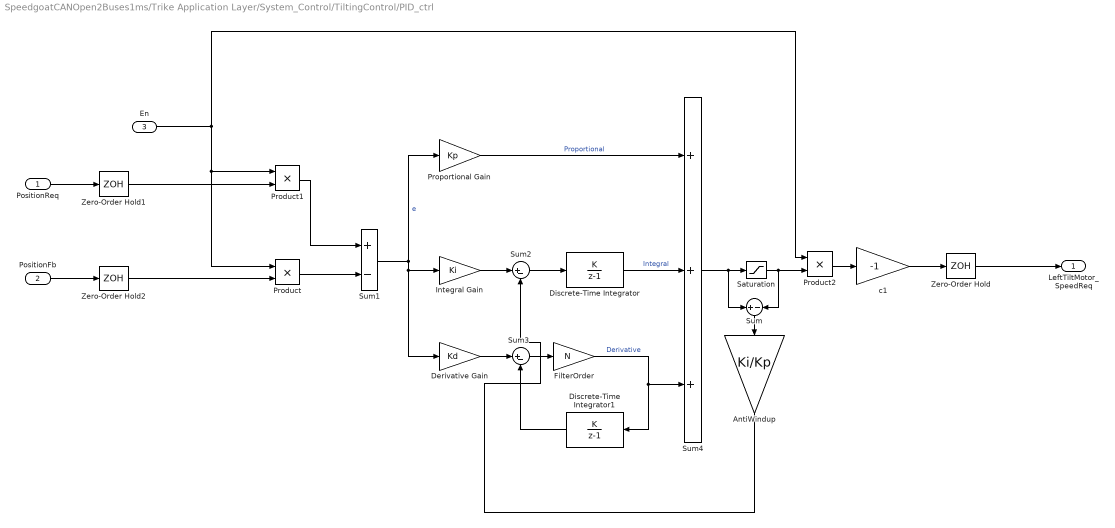
== system SpeedgoatCANOpen2Buses1ms/Trike Application Layer/System_Control/TiltingControl/PID_ctrl ==
  PositionReq : Inport
  PositionFb : Inport  Port=2
  En : Inport  Port=3
  AntiWindup : Gain  Gain=Ki/Kp  SaturateOnIntegerOverflow=on  OutDataTypeStr=Inherit: Same as input  ParamDataTypeStr=Inherit: Same as input
  Derivative Gain : Gain  Gain=Kd  SaturateOnIntegerOverflow=on  OutDataTypeStr=Inherit: Same as input  ParamDataTypeStr=Inherit: Same as input
  Discrete-Time Integrator : DiscreteIntegrator  IntegratorMethod=Accumulation: Forward Euler  gainval=Ts/5  SampleTime=-1  ICPrevOutput=DiscIntNeverNeededParam  ICPrevScaledInput=DiscIntNeverNeededParam
  Discrete-Time Integrator1 : DiscreteIntegrator  IntegratorMethod=Accumulation: Forward Euler  gainval=Ts/5  SampleTime=-1  ICPrevOutput=DiscIntNeverNeededParam  ICPrevScaledInput=DiscIntNeverNeededParam
  FilterOrder : Gain  Gain=N  SaturateOnIntegerOverflow=on  OutDataTypeStr=Inherit: Same as input  ParamDataTypeStr=Inherit: Same as input
  Integral Gain : Gain  Gain=Ki  SaturateOnIntegerOverflow=on  OutDataTypeStr=Inherit: Same as input  ParamDataTypeStr=Inherit: Same as input
  Product : Product
  Product1 : Product
  Product2 : Product
  Proportional Gain : Gain  Gain=Kp  SaturateOnIntegerOverflow=on  OutDataTypeStr=Inherit: Same as input  ParamDataTypeStr=Inherit: Same as input
  Saturation : Saturate  UpperLimit=Req_lim  LowerLimit=-Req_lim
  Sum : Sum  Inputs=+|-
  Sum1 : Sum  Inputs=+-  SaturateOnIntegerOverflow=on  InputSameDT=on  OutDataTypeStr=Inherit: Same as first input
  Sum2 : Sum  Inputs=|+-
  Sum3 : Sum  Inputs=|+-
  Sum4 : Sum  Inputs=+++  SaturateOnIntegerOverflow=on  InputSameDT=on  OutDataTypeStr=Inherit: Same as first input
  Zero-Order Hold : ZeroOrderHold  SampleTime=Ts
  Zero-Order Hold1 : ZeroOrderHold  SampleTime=Ts
  Zero-Order Hold2 : ZeroOrderHold  SampleTime=Ts
  c1 : Gain  Gain=-1
  LeftTiltMotor_SpeedReq : Outport  VectorParamsAs1DForOutWhenUnconnected=on
  wires:
  Saturation/1 -> Product2/2, Sum/2
  AntiWindup/1 -> Sum2/2
  Sum2/1 -> Discrete-Time Integrator/1
  Sum4/1 -> Sum/1, Saturation/1
  Proportional Gain/1 -> Sum4/1  "Proportional"
  Integral Gain/1 -> Sum2/1
  Sum/1 -> AntiWindup/1
  Discrete-Time Integrator/1 -> Sum4/2  "Integral"
  PositionFb/1 -> Zero-Order Hold2/1
  Product1/1 -> Sum1/1
  Product/1 -> Sum1/2
  En/1 -> Product2/1, Product/1, Product1/1
  PositionReq/1 -> Zero-Order Hold1/1
  Product2/1 -> c1/1
  Derivative Gain/1 -> Sum3/1
  Discrete-Time Integrator1/1 -> Sum3/2
  Sum1/1 -> Proportional Gain/1, Derivative Gain/1, Integral Gain/1  "e"
  Sum3/1 -> FilterOrder/1
  FilterOrder/1 -> Sum4/3, Discrete-Time Integrator1/1  "Derivative"
  c1/1 -> Zero-Order Hold/1
  Zero-Order Hold/1 -> LeftTiltMotor_SpeedReq/1
  Zero-Order Hold1/1 -> Product1/2
  Zero-Order Hold2/1 -> Product/2

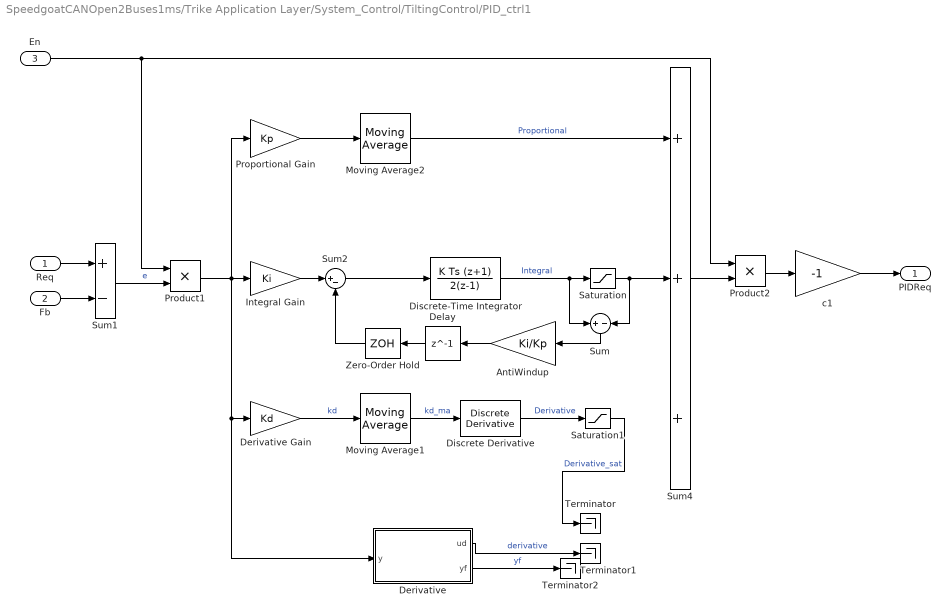
== system SpeedgoatCANOpen2Buses1ms/Trike Application Layer/System_Control/TiltingControl/PID_ctrl1 ==
  Req : Inport
  Fb : Inport  Port=2
  En : Inport  Port=3
  AntiWindup : Gain  Gain=Ki/Kp  SaturateOnIntegerOverflow=on  OutDataTypeStr=Inherit: Same as input  ParamDataTypeStr=Inherit: Same as input
  Delay : Delay  DelayLength=1  SampleTime=0.005
  Derivative : MATLAB Function  TreatAsAtomicUnit=on  SystemSampleTime=0.005
      settings: MinAlgLoopOccurrences=on
  Derivative Gain : Gain  Gain=Kd  SaturateOnIntegerOverflow=on  OutDataTypeStr=Inherit: Same as input  ParamDataTypeStr=Inherit: Same as input
  Discrete Derivative : simulink/Discrete/Discrete Derivative  gainval=1.0  ICPrevScaledInput=0.0  OutMin=[]  OutMax=[]  OutDataType=fixdt(1, 16)  OutScaling=2^-10  DoSatur=off
  Discrete-Time Integrator : DiscreteIntegrator  IntegratorMethod=Integration: Trapezoidal  gainval=1  SampleTime=Ts  ICPrevOutput=DiscIntNeverNeededParam  ICPrevScaledInput=DiscIntNeverNeededParam
  Integral Gain : Gain  Gain=Ki  SaturateOnIntegerOverflow=on  OutDataTypeStr=Inherit: Same as input  ParamDataTypeStr=Inherit: Same as input
  Moving Average1 : dspstat3/Moving Average  Method=Sliding window  ForgettingFactorPort=off  SpecifyWindowLength=on  WindowLength=N  ForgettingFactor=0.9  SimulateUsing=Code generation
  Moving Average2 : dspstat3/Moving Average  Method=Sliding window  ForgettingFactorPort=off  SpecifyWindowLength=on  WindowLength=1  ForgettingFactor=0.9  SimulateUsing=Code generation
  Product1 : Product
  Product2 : Product
  Proportional Gain : Gain  Gain=Kp  SaturateOnIntegerOverflow=on  OutDataTypeStr=Inherit: Same as input  ParamDataTypeStr=Inherit: Same as input
  Saturation : Saturate  UpperLimit=Req_lim  LowerLimit=-Req_lim
  Saturation1 : Saturate  UpperLimit=Req_lim  LowerLimit=-Req_lim
  Sum : Sum  Inputs=+|-
  Sum1 : Sum  Inputs=+-  SaturateOnIntegerOverflow=on  InputSameDT=on  OutDataTypeStr=Inherit: Same as first input
  Sum2 : Sum  Inputs=|+-
  Sum4 : Sum  Inputs=+++  SaturateOnIntegerOverflow=on  InputSameDT=on  OutDataTypeStr=Inherit: Same as first input
  Terminator : Terminator
  Terminator1 : Terminator
  Terminator2 : Terminator
  Zero-Order Hold : ZeroOrderHold  SampleTime=0.005
  c1 : Gain  Gain=-1
  PIDReq : Outport  VectorParamsAs1DForOutWhenUnconnected=on
  wires:
  c1/1 -> PIDReq/1
  Derivative Gain/1 -> Moving Average1/1  "kd"
  Fb/1 -> Sum1/2
  Req/1 -> Sum1/1
  Discrete-Time Integrator/1 -> Saturation/1, Sum/1  "Integral"
  Sum/1 -> AntiWindup/1
  Integral Gain/1 -> Sum2/1
  Proportional Gain/1 -> Moving Average2/1
  Sum2/1 -> Discrete-Time Integrator/1
  Saturation/1 -> Sum4/2, Sum/2
  AntiWindup/1 -> Delay/1
  Sum4/1 -> Product2/2
  Sum1/1 -> Product1/2  "e"
  Discrete Derivative/1 -> Saturation1/1  "Derivative"
  Saturation1/1 -> Terminator/1  "Derivative_sat"
  En/1 -> Product1/1, Product2/1
  Product2/1 -> c1/1
  Product1/1 -> Proportional Gain/1, Derivative/1(y), Derivative Gain/1, Integral Gain/1
  Delay/1 -> Zero-Order Hold/1
  Zero-Order Hold/1 -> Sum2/2
  Moving Average2/1 -> Sum4/1  "Proportional"
  Moving Average1/1 -> Discrete Derivative/1  "kd_ma"
  Derivative/1(ud) -> Terminator1/1  "derivative"
  Derivative/2(yf) -> Terminator2/1  "yf"

== system SpeedgoatCANOpen2Buses1ms/Trike Application Layer/System_Control/TiltingControl/TiltingController ==
  "PosRef [m] " : Inport
  PosFb [m] : Inport  Port=2
  "En " : Inport  Port=3
  PID_Clasic_V1 : Subsystem  VariantControl=V1
  PID_Incremental_V1 : Subsystem  VariantControl=V2
  " LTilt SpeedRef" : Outport
  " RTilt SpeedRef" : Outport  Port=2

== system SpeedgoatCANOpen2Buses1ms/Trike Application Layer/System_Control/TiltingControl/TiltingController/PID_Clasic_V1 ==
  PosRef [m] : Inport
  PosFb [m] : Inport  Port=2
  En : Inport  Port=3
  PID_ctrl : Subsystem  mask{Kp=150, Ki=0, Kd=0, Ts=0.001, N=1, FF_En=0, Req_lim=2}
      mask prompts: N "FilterOrder"; FF_En "FeedForward En"; Req_lim "Req_sat"
  " LTilt SpeedRef" : Outport
  " RTilt SpeedRef" : Outport  Port=2
  wires:
  En/1 -> PID_ctrl/3(En)
  PID_ctrl/2(RTilt Speed) -> " RTilt SpeedRef"/1  "RTilt CurrenRef"
  PID_ctrl/1(LTilt Speed) -> " LTilt SpeedRef"/1  "LTilt CurrentRef"
  PosFb [m]/1 -> PID_ctrl/2(PosFb)
  PosRef [m]/1 -> PID_ctrl/1(PosRef)

== system SpeedgoatCANOpen2Buses1ms/Trike Application Layer/System_Control/TiltingControl/TiltingController/PID_Incremental_V1 ==
  PosRef [m] : Inport
  PosFb [m] : Inport  Port=2
  En : Inport  Port=3
  PI_incremental Tilting Controller : MATLAB Function  TreatAsAtomicUnit=on  SystemSampleTime=5e-3
  Terminator1 : Terminator
  Terminator2 : Terminator
  Terminator7 : Terminator
  " LTilt SpeedRef" : Outport
  " RTilt SpeedRef" : Outport  Port=2
  wires:
  En/1 -> PI_incremental Tilting Controller/3(En)
  PI_incremental Tilting Controller/2(RTiltCurrRef) -> " RTilt SpeedRef"/1  "RTilt CurrenRef"
  PI_incremental Tilting Controller/1(LTiltCurrRef) -> " LTilt SpeedRef"/1  "LTilt CurrentRef"
  PosFb [m]/1 -> PI_incremental Tilting Controller/2(Pos)
  PosRef [m]/1 -> PI_incremental Tilting Controller/1(PosRef)
  PI_incremental Tilting Controller/3(up) -> Terminator7/1  "up"
  PI_incremental Tilting Controller/4(ui) -> Terminator1/1  "ui"
  PI_incremental Tilting Controller/5(ud) -> Terminator2/1  "ud"

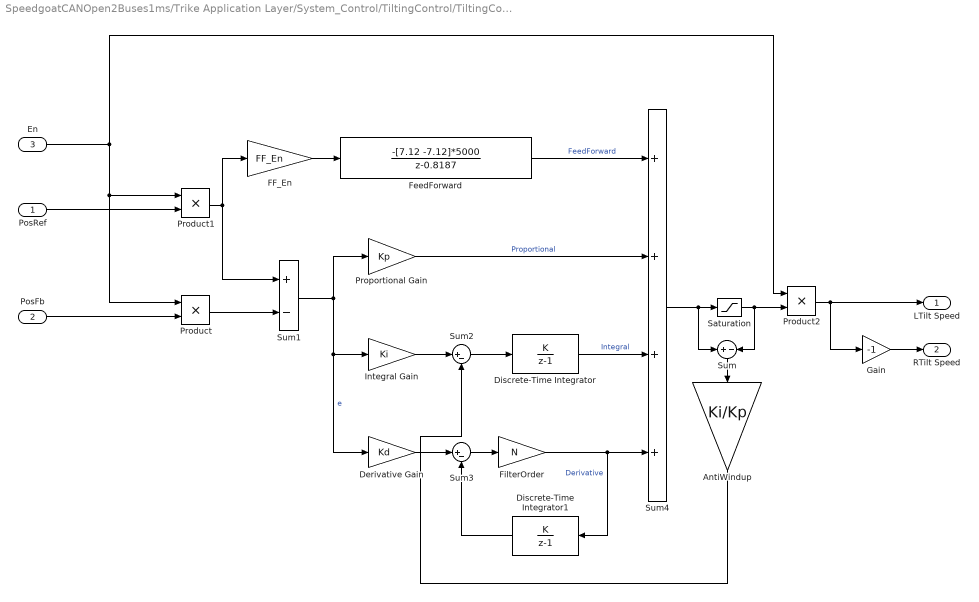
== system SpeedgoatCANOpen2Buses1ms/Trike Application Layer/System_Control/TiltingControl/TiltingController/PID_Clasic_V1/PID_ctrl ==
  PosRef : Inport
  PosFb : Inport  Port=2
  En : Inport  Port=3
  AntiWindup : Gain  Gain=Ki/Kp  SaturateOnIntegerOverflow=on  OutDataTypeStr=Inherit: Same as input  ParamDataTypeStr=Inherit: Same as input
  Derivative Gain : Gain  Gain=Kd  SaturateOnIntegerOverflow=on  OutDataTypeStr=Inherit: Same as input  ParamDataTypeStr=Inherit: Same as input
  Discrete-Time Integrator : DiscreteIntegrator  IntegratorMethod=Accumulation: Forward Euler  gainval=Ts/5  SampleTime=-1  ICPrevOutput=DiscIntNeverNeededParam  ICPrevScaledInput=DiscIntNeverNeededParam
  Discrete-Time Integrator1 : DiscreteIntegrator  IntegratorMethod=Accumulation: Forward Euler  gainval=Ts/5  SampleTime=-1  ICPrevOutput=DiscIntNeverNeededParam  ICPrevScaledInput=DiscIntNeverNeededParam
  FF_En : Gain  Gain=FF_En  SaturateOnIntegerOverflow=on  OutDataTypeStr=Inherit: Same as input  ParamDataTypeStr=Inherit: Same as input
  FeedForward : DiscreteTransferFcn  Numerator=-[7.12 -7.12]*5000  Denominator=[1 -0.8187]  SampleTime=Ts/5
  FilterOrder : Gain  Gain=N  SaturateOnIntegerOverflow=on  OutDataTypeStr=Inherit: Same as input  ParamDataTypeStr=Inherit: Same as input
  Gain : Gain  Gain=-1
  Integral Gain : Gain  Gain=Ki  SaturateOnIntegerOverflow=on  OutDataTypeStr=Inherit: Same as input  ParamDataTypeStr=Inherit: Same as input
  Product : Product
  Product1 : Product
  Product2 : Product
  Proportional Gain : Gain  Gain=Kp  SaturateOnIntegerOverflow=on  OutDataTypeStr=Inherit: Same as input  ParamDataTypeStr=Inherit: Same as input
  Saturation : Saturate  UpperLimit=Req_lim  LowerLimit=-Req_lim
  Sum : Sum  Inputs=+|-
  Sum1 : Sum  Inputs=+-  SaturateOnIntegerOverflow=on  InputSameDT=on  OutDataTypeStr=Inherit: Same as first input
  Sum2 : Sum  Inputs=|+-
  Sum3 : Sum  Inputs=|+-
  Sum4 : Sum  Inputs=++++  SaturateOnIntegerOverflow=on  InputSameDT=on  OutDataTypeStr=Inherit: Same as first input
  LTilt Speed : Outport  VectorParamsAs1DForOutWhenUnconnected=on
  RTilt Speed : Outport  Port=2  VectorParamsAs1DForOutWhenUnconnected=on
  wires:
  Saturation/1 -> Product2/2, Sum/2
  AntiWindup/1 -> Sum2/2
  Sum2/1 -> Discrete-Time Integrator/1
  Sum4/1 -> Sum/1, Saturation/1
  FeedForward/1 -> Sum4/1  "FeedForward"
  Proportional Gain/1 -> Sum4/2  "Proportional"
  Integral Gain/1 -> Sum2/1
  Sum/1 -> AntiWindup/1
  Discrete-Time Integrator/1 -> Sum4/3  "Integral"
  PosFb/1 -> Product/2
  Product1/1 -> Sum1/1, FF_En/1
  Product/1 -> Sum1/2
  En/1 -> Product2/1, Product/1, Product1/1
  PosRef/1 -> Product1/2
  Product2/1 -> Gain/1, LTilt Speed/1
  Gain/1 -> RTilt Speed/1
  Derivative Gain/1 -> Sum3/1
  Discrete-Time Integrator1/1 -> Sum3/2
  Sum1/1 -> Proportional Gain/1, Derivative Gain/1, Integral Gain/1  "e"
  Sum3/1 -> FilterOrder/1
  FilterOrder/1 -> Sum4/4, Discrete-Time Integrator1/1  "Derivative"
  FF_En/1 -> FeedForward/1

== stateflow chart SpeedgoatCANOpen2Buses1ms/Trike Application Layer/System_Init/TiltingRight_DunkMotor_Init/DunkB_TiltRight_Init_CurrentMode ==
  state Init
    entry:
    ClearError       = 0;
    DeviceMode   = 0;
    BrakeCtrl        = 0;
    PowerEnable = 0;
    aux                 = 0;
    InitStatus        = 0;
  state Clear_Error
    du:
    ClearError = 1;
    aux            = aux + 1;
    InitStatus   = 0;
  state Wait
    en:
    BrakeCtrl = 2;
    aux          = aux + 1;
    InitStatus = 0;
  state SetCurrentMode
    du:
    DeviceMode  = 2;%2 current
    PowerEnable = 1;
    InitStatus       = 1;
  (default) -> Init
  Init -> Clear_Error : %[ButtonStatus == 1 ||...
      | %  ReadError ~= 1]
  Clear_Error -> Wait : [aux > 40000]{aux = 0;}
  (junction 262) -> Init
  Wait -> Wait [order 1] : [aux < 20 && ReadError == 1]
  Wait -> (junction 262) [order 3] : [ReadError ~= 1]
  (junction 263) -> (junction 262)
  Wait -> SetCurrentMode [order 2] : [aux >= 20 && ReadError == 1]{aux = 0;}
  SetCurrentMode -> (junction 263) : [ReadError ~= 1]
  data: ButtonStatus input single; ClearError output single; DeviceMode output single; BrakeCtrl output single; ReadError input single; aux2 local single; aux local single; PowerEnable output single; InitStatus output single

== stateflow chart SpeedgoatCANOpen2Buses1ms/Trike Application Layer/System_Init/TiltingLeft_DunkMotor_Init/DunkC_TiltLeft_Init_CurrentMode ==
  state Init
    entry:
    ClearError       = 0;
    DeviceMode   = 0;
    BrakeCtrl        = 0;
    PowerEnable = 0;
    aux                 = 0;
    InitStatus        = 0;
  state Clear_Error
    du:
    ClearError = 1;
    aux            = aux + 1;
    InitStatus   = 0;
  state Wait
    en:
    BrakeCtrl = 2;
    aux          = aux + 1;
    InitStatus = 0;
  state SetCurrentMode
    du:
    DeviceMode  = 3; % 3 speed
    PowerEnable = 1;
    InitStatus       = 1;
  (default) -> Init
  Init -> Clear_Error : %[ButtonStatus == 1 ||...
      | %  ReadError ~= 1]
  Clear_Error -> Wait : [aux > 40000]{aux = 0;}
  (junction 253) -> Init
  Wait -> Wait [order 1] : [aux < 20 && ReadError == 1]
  Wait -> (junction 253) [order 3] : [ReadError ~= 1]
  (junction 254) -> (junction 253)
  Wait -> SetCurrentMode [order 2] : [aux >= 20 && ReadError == 1]{aux = 0;}
  SetCurrentMode -> (junction 254) : [ReadError ~= 1]
  data: ButtonStatus input single; ClearError output single; DeviceMode output single; BrakeCtrl output single; ReadError input single; aux2 local single; aux local single; PowerEnable output single; InitStatus output single

== stateflow chart SpeedgoatCANOpen2Buses1ms/Trike Application Layer/System_Init/Brakes_DunkMotor_Init/DunkD_Brake_Init_CurrentMode ==
  state Init
    entry:
    ClearError       = 0;
    DeviceMode   = 0;
    BrakeCtrl        = 2; %0
    PowerEnable = 0;
    aux                 = 0;
    InitStatus        = 0;
    BrakesMotor_CurrentInit = 0;
  state Clear_Error
    du:
    ClearError = 1;
    aux            = aux + 1;
    InitStatus   = 0;
  state Wait
    en:
    BrakeCtrl = 2;
    aux          = aux + 1;
    InitStatus = 0;
  state SetCurrentMode
    du:
    DeviceMode       = 2;
    PowerEnable      = 1;
    InitStatus            = 1;
    BrakesMotor_CurrentInit = 11000;
    aux                     = aux + 1;
  state SetCurrentMode1
    du:
    InitStatus            = 1;
    BrakeCtrl            = 2;%0
    BrakesMotor_CurrentInit = 0;
  (default) -> Init
  Init -> Clear_Error : %[ButtonStatus == 1 ||...
      | % ReadError ~= 1]
  Clear_Error -> Wait : [aux>40000]{aux = 0;}
  (junction 259) -> Init
  Wait -> Wait [order 1] : [aux < 20  && ReadError == 1]
  Wait -> (junction 259) [order 3] : [ReadError ~= 1]
  (junction 260) -> (junction 259)
  Wait -> SetCurrentMode [order 2] : [aux >= 20 && ReadError == 1]{aux = 0;}
  SetCurrentMode -> (junction 260) [order 1] : [ReadError ~= 1]
  (junction 261) -> (junction 260)
  SetCurrentMode -> SetCurrentMode1 [order 2] : [aux > 10000]
  SetCurrentMode1 -> (junction 261) : [ReadError ~= 1]
  data: ButtonStatus input single; ClearError output single; DeviceMode output single; BrakeCtrl output single; ReadError input single; aux2 local single; aux local single; PowerEnable output single; BrakesMotor_CurrentInit output single [-12000..12000]; InitStatus output single
